simulink model "Kenematics_and_IKenematics_Func_Simulink"  (R2021a)
settings: Solver=VariableStepAuto  StartTime=0.0  StopTime=10.0  RelTol=1e-3
settings Model: Creator=WU  LastModifiedBy=WU

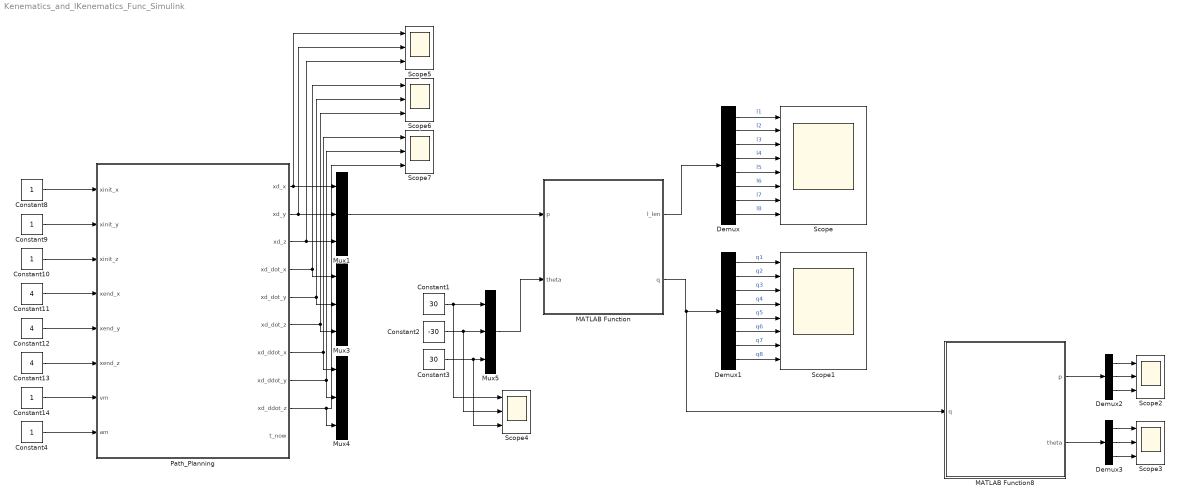
== system Kenematics_and_IKenematics_Func_Simulink ==
  Constant1 : Constant  Value=30  VectorParams1D=off
  Constant{4,9..10,14} (4 alike) : Constant
  Constant11 : Constant  Value=4
  Constant12 : Constant  Value=4
  Constant13 : Constant  Value=4
  Constant2 : Constant  Value=-30
  Constant3 : Constant  Value=30
  Constant8 : Constant  VectorParams1D=off
  Demux : Demux  Outputs=8
  Demux1 : Demux  Outputs=8
  Demux2 : Demux  Outputs=3
      settings: DisplayOption=none
  Demux3 : Demux  Outputs=3
      settings: DisplayOption=none
  MATLAB Function : MATLAB Function  TreatAsAtomicUnit=on
  MATLAB Function8 : MATLAB Function  TreatAsAtomicUnit=on
  Mux{1,3..5} (4 alike) : Mux  Inputs=3
  Path_Planning : Subsystem
  Scope : Scope  NumInputPorts=8
  Scope1 : Scope  NumInputPorts=8
  Scope{2..7} (6 alike) : Scope  NumInputPorts=3
  wires:
  Constant4/1 -> Path_Planning/8(am)
  Path_Planning/9(xd_ddot_z) -> Scope7/3, Mux4/3
  Constant13/1 -> Path_Planning/6(xend_z)
  Path_Planning/5(xd_dot_y) -> Scope6/2, Mux3/2
  Constant9/1 -> Path_Planning/2(xinit_y)
  Constant8/1 -> Path_Planning/1(xinit_x)
  Constant12/1 -> Path_Planning/5(xend_y)
  Path_Planning/7(xd_ddot_x) -> Scope7/1, Mux4/1
  Constant11/1 -> Path_Planning/4(xend_x)
  Path_Planning/3(xd_z) -> Scope5/3, Mux1/3
  Constant14/1 -> Path_Planning/7(vm)
  Path_Planning/4(xd_dot_x) -> Scope6/1, Mux3/1
  Path_Planning/8(xd_ddot_y) -> Scope7/2, Mux4/2
  Path_Planning/2(xd_y) -> Scope5/2, Mux1/2
  Constant10/1 -> Path_Planning/3(xinit_z)
  Path_Planning/1(xd_x) -> Scope5/1, Mux1/1
  Path_Planning/6(xd_dot_z) -> Scope6/3, Mux3/3
  Mux1/1 -> MATLAB Function/1(p)
  Constant2/1 -> Scope4/2, Mux5/2
  Constant1/1 -> Scope4/1, Mux5/1
  Constant3/1 -> Scope4/3, Mux5/3
  Mux5/1 -> MATLAB Function/2(theta)
  MATLAB Function/1(l_len) -> Demux/1
  Demux/1 -> Scope/1  "l1"
  Demux/2 -> Scope/2  "l2"
  Demux/3 -> Scope/3  "l3"
  Demux/4 -> Scope/4  "l4"
  Demux/5 -> Scope/5  "l5"
  Demux/6 -> Scope/6  "l6"
  Demux/8 -> Scope/8  "l8"
  Demux/7 -> Scope/7  "l7"
  Demux1/1 -> Scope1/1  "q1"
  Demux1/4 -> Scope1/4  "q4"
  Demux1/5 -> Scope1/5  "q5"
  Demux1/8 -> Scope1/8  "q8"
  Demux1/2 -> Scope1/2  "q2"
  Demux1/3 -> Scope1/3  "q3"
  Demux1/7 -> Scope1/7  "q7"
  Demux1/6 -> Scope1/6  "q6"
  MATLAB Function/2(q) -> MATLAB Function8/1(q), Demux1/1
  MATLAB Function8/1(p) -> Demux2/1
  MATLAB Function8/2(theta) -> Demux3/1
  Demux2/1 -> Scope2/1
  Demux2/2 -> Scope2/2
  Demux2/3 -> Scope2/3
  Demux3/1 -> Scope3/1
  Demux3/2 -> Scope3/2
  Demux3/3 -> Scope3/3

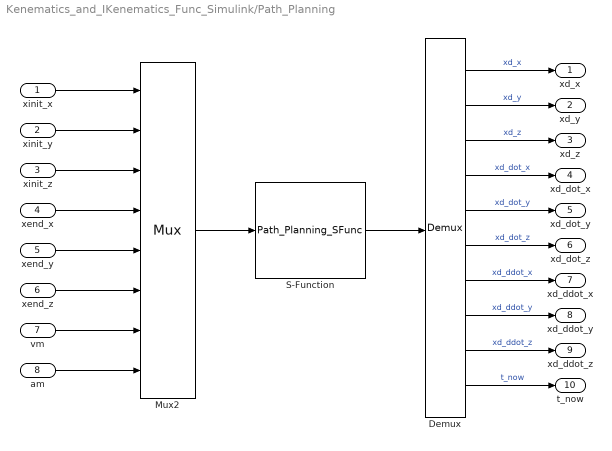
== system Kenematics_and_IKenematics_Func_Simulink/Path_Planning ==
  xinit_x : Inport
  xinit_y : Inport  Port=2
  xinit_z : Inport  Port=3
  xend_x : Inport  Port=4
  xend_y : Inport  Port=5
  xend_z : Inport  Port=6
  vm : Inport  Port=7
  am : Inport  Port=8
  Demux : Demux  Outputs=10
      settings: DisplayOption=none
  Mux2 : Mux  Inputs=8
  S-Function : S-Function  FunctionName=Path_Planning_SFunc  SFunctionDeploymentMode=off  EnableBusSupport=off
  xd_x : Outport
  xd_y : Outport  Port=2
  xd_z : Outport  Port=3
  xd_dot_x : Outport  Port=4
  xd_dot_y : Outport  Port=5
  xd_dot_z : Outport  Port=6
  xd_ddot_x : Outport  Port=7
  xd_ddot_y : Outport  Port=8
  xd_ddot_z : Outport  Port=9
  t_now : Outport  Port=10
  wires:
  Demux/7 -> xd_ddot_x/1  "xd_ddot_x"
  vm/1 -> Mux2/7
  xinit_y/1 -> Mux2/2
  Demux/1 -> xd_x/1  "xd_x"
  Demux/4 -> xd_dot_x/1  "xd_dot_x"
  Demux/5 -> xd_dot_y/1  "xd_dot_y"
  Demux/9 -> xd_ddot_z/1  "xd_ddot_z"
  Demux/8 -> xd_ddot_y/1  "xd_ddot_y"
  Demux/3 -> xd_z/1  "xd_z"
  Demux/6 -> xd_dot_z/1  "xd_dot_z"
  Demux/2 -> xd_y/1  "xd_y"
  xend_y/1 -> Mux2/5
  Mux2/1 -> S-Function/1
  S-Function/1 -> Demux/1
  xend_z/1 -> Mux2/6
  xend_x/1 -> Mux2/4
  xinit_z/1 -> Mux2/3
  xinit_x/1 -> Mux2/1
  am/1 -> Mux2/8
  Demux/10 -> t_now/1  "t_now"

== matlab function Kenematics_and_IKenematics_Func_Simulink/MATLAB Function8 ==
  data: q input; p output; theta output
function [p,theta] = ForwardKenamatics_Func(q)
%*********************************************************
%使用LM法求解运动学正解，迭代起点在base内部空间任意选择；
%输入参数：L 绳索长度构成的行向量；
%输出参数：solution 动平台的位姿向量
%         k 迭代次数
%         minF 误差F的最终值
%*********************************************************
%%
%base/plateform的基本数据：
%base:L*W*H=15*11*6
%drawing points在O-XYZ中表示：

A=zeros(3,8);
Bp=zeros(3,8);

A(1:3,1)=[-7.5 -5.5 6]';
A(1:3,2)=[-7.5 -5.5 6];
A(1:3,3)=[-7.5 5.5 6]';
A(1:3,4)=[-7.5 5.5 6]';
A(1:3,5)=[7.5 5.5 6]';
A(1:3,6)=[7.5 5.5 6];
A(1:3,7)=[7.5 -5.5 6];
A(1:3,8)=[7.5 -5.5 6]';
%plateform:l*w*h=1*1*1
%attach points在P-XpYpZp中表示：
Bp(1:3,1)=[0.5 -0.5 0]';
Bp(1:3,2)=[-0.5 0.5 1]';
Bp(1:3,3)=[-0.5 -0.5 0]';
Bp(1:3,4)=[0.5 0.5 1]';
Bp(1:3,5)=[-0.5 0.5 0]';
Bp(1:3,6)=[0.5 -0.5 1]';
Bp(1:3,7)=[0.5 0.5 0]';
Bp(1:3,8)=[-0.5 -0.5 1]';

%%
%约束函数向量为vector_f；目标函数为F;
%采用《methods for non-linear least squares problems》中表述：F=1/2*sum(fi(x)^2)=1/2*(vector_f'*vector_f)
l=0.0225*q';
length_given=l;
%下面为LM法参数：
%设置stop criteria:
epsilon1=1.0e-8;
epsilon2=1.0e-8;
%设置迭代次数上限：
k_max=100;
%当前迭代次数：
k=0;
%设置初始迭代位置:设置为固定平台中心位置
%pose_position_angle=[x y z angle_x angle_y angle_z]
pose_position_angle=[0 0 1 0 0 0];
%u的增长因子v
v=2;
%结束标志
found=false;

%% 统计时间的开始
%LM算法计算开始：
jacobian_f=Jaco(pose_position_angle,A,Bp);
A_matrix=jacobian_f'*jacobian_f;
vector_f=FunctionVector_f(pose_position_angle,A,Bp,length_given);
g=jacobian_f'*vector_f;

if norm(g)<=epsilon1
    found=true;
end

%设置初始damped parameter u
tau=1.0e-3;
u=tau*max([A_matrix(1,1),A_matrix(2,2),A_matrix(3,3),A_matrix(4,4),A_matrix(5,5),A_matrix(6,6)]);

while(found==false)&&(k<=k_max)
    k=k+1;
    %解的迭代方向及步长
    h_lm=(A_matrix+u*eye(6,6))\(-1*g);
    %h_lm=inv(A_matrix+u*eye(6,6))*(-1*g);
    if norm(h_lm)<=(epsilon2*(norm(pose_position_angle))+epsilon2)
        found=true;
    else
        pose_position_angle_new=pose_position_angle+h_lm';
        vector_f_new=FunctionVector_f(pose_position_angle_new,A,Bp,length_given);
        %计算更新指标Q
        Q=Q_criteria(vector_f,vector_f_new,h_lm,u,g);
        
        if Q>0
            
            pose_position_angle=pose_position_angle_new;
            
            jacobian_f=Jaco(pose_position_angle,A,Bp);
            A_matrix=jacobian_f'*jacobian_f;
            vector_f=FunctionVector_f(pose_position_angle,A,Bp,length_given);
            g=jacobian_f'*vector_f;
            
            if norm(g)<=epsilon1
                found=true;
            end
            u=u*max([1/3, 1, 1-(2*Q-1)^3]);
            v=2;
        else
            u=u*v;
            v=2*v;
        end
        
    end
    
    
end

solution=pose_position_angle';
p=solution(1:3,1);
theta=solution(4:6,1)/pi*(180);

end

== matlab function Kenematics_and_IKenematics_Func_Simulink/MATLAB Function ==
  data: p input; l_len output; theta input; q output
function [l_len,q]  = InverseKenematics_Func(p,theta)
%UNTITLED3 求解CDPRs的逆运动学解
%   Detailed explanation goes here
x=theta(1);
y=theta(2);
z=theta(3);
Rxyz=Theta2RotationMatrix_Func(x,y,z);
%% CoGiRo的参数 8绳索6自由度的CDPRs
% ai的定义
a1=[-7.5 -5.5 6]';
a2=[-7.5 -5.5 6]';
a3=[-7.5 5.5 6]';
a4=[-7.5 5.5 6]';
a5=[7.5 5.5 6]';
a6=[7.5 5.5 6]';
a7=[7.5 -5.5 6]';
a8=[7.5 -5.5 6]';
% bi的定义
b1=[0.5 -0.5 0]';
b2=[-0.5 0.5 1]';
b3=[-0.5 -0.5 0]';
b4=[0.5 0.5 1]';
b5=[-0.5 0.5 0]';
b6=[0.5 -0.5 1]';
b7=[0.5 0.5 0]';
b8=[-0.5 -0.5 1]';
%% 计算li=ai-xp-Rbi
l1=a1-p-Rxyz*b1;
l2=a2-p-Rxyz*b2;
l3=a3-p-Rxyz*b3;
l4=a4-p-Rxyz*b4;
l5=a5-p-Rxyz*b5;
l6=a6-p-Rxyz*b6;
l7=a7-p-Rxyz*b7;
l8=a8-p-Rxyz*b8;
% 求绳索向量的模长
l1_len=norm(l1);
l2_len=norm(l2);
l3_len=norm(l3);
l4_len=norm(l4);
l5_len=norm(l5);
l6_len=norm(l6);
l7_len=norm(l7);
l8_len=norm(l8);
% l=[l1 l2 l3 l4 l5 l6 l7 l8]';
l_len=[l1_len l2_len l3_len l4_len l5_len l6_len l7_len l8_len]';
q=l_len./0.0225;
end
